simulink model "GPCA_INFUSION_MGR"  (Simulink 8.5)
settings: Solver=ode45  StartTime=0.0  StopTime=10.0  RelTol=1e-3
libraries: simulink x4
settings Model: Creator=bourbouh  LastModifiedBy=Teme
settings DataIOCC: LimitDataPoints=off  SaveFormat=Dataset  SignalLoggingSaveFormat=Dataset
settings OptimizationCC: ExpressionDepthLimit=128
settings DebuggingCC: UnderspecifiedInitializationDetection=Simplified  MergeDetectMultiDrivingBlocksExec=error  FcnCallInpInsideContextMsg=EnableAllAsError  StateNameClashWarn=none
settings HardwareCC: ProdBitPerInt=16  ProdBitPerPointer=16  ProdIntDivRoundTo=Zero  ProdWordSize=8  ProdShiftRightIntArith=off  ProdHWDeviceType=Intel->8051 Compatible  TargetBitPerPointer=64  TargetLargestAtomicFloat=Float  TargetIntDivRoundTo=Zero  TargetEndianess=LittleEndian  TargetWordSize=64  TargetHWDeviceType=Intel->x86-64 (Windows64)  ProdEqTarget=off
settings ModelReferenceCC: PropagateSignalLabelsOutOfModel=on
settings GRTTargetCC: CombineOutputUpdateFcns=on  GRTInterface=off
settings ConfigComp: CovMetricSettings=dw  CovHtmlReporting=on  CovSaveCumulativeToWorkspaceVar=on  CovSaveSingleToWorkspaceVar=on  CovExternalEMLEnable=off

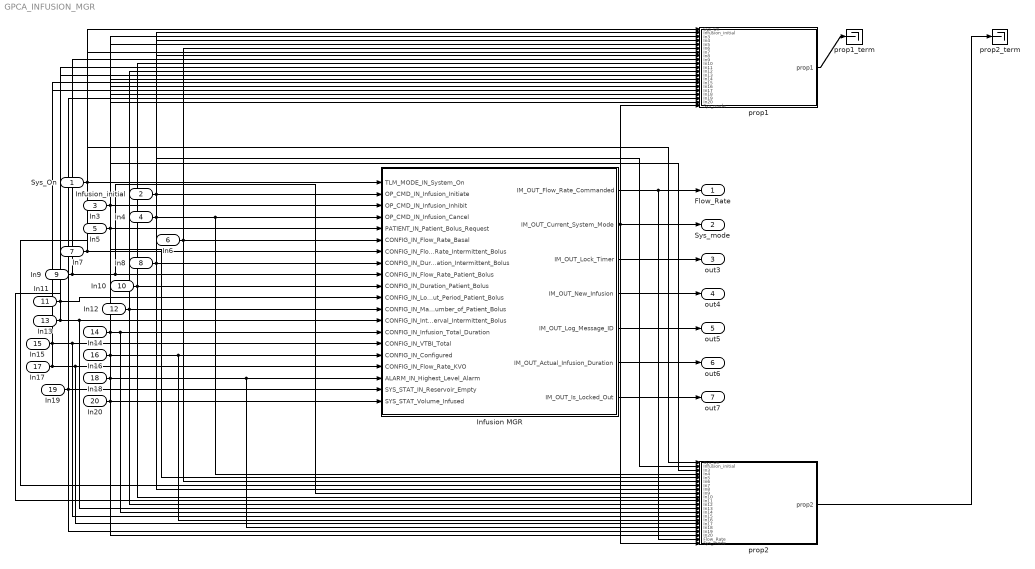
== system GPCA_INFUSION_MGR ==
  Sys_On : Inport
  Infusion_initial : Inport  Port=2
  In3 : Inport  Port=3
  In4 : Inport  Port=4
  In5 : Inport  Port=5
  In6 : Inport  Port=6
  In7 : Inport  Port=7
  In8 : Inport  Port=8
  In9 : Inport  Port=9
  In10 : Inport  Port=10
  In11 : Inport  Port=11
  In12 : Inport  Port=12
  In13 : Inport  Port=13
  In14 : Inport  Port=14
  In15 : Inport  Port=15
  In16 : Inport  Port=16
  In17 : Inport  Port=17
  In18 : Inport  Port=18
  In19 : Inport  Port=19
  In20 : Inport  Port=20
  Infusion MGR : Stateflow chart  TreatAsAtomicUnit=on
  prop1 : Subsystem  TreatAsAtomicUnit=on  mask(Observer){AnnotationType=ensures, ObserverType=[]}
      mask prompts: AnnotationType "Type of annotation (pre/post...)"; ObserverType "Observer type"
      mask help:
      | Set an observer for the system.
      | The annotation type parameter sets the type of observer:
      | - requires : pre-condition
      | - ensures : post-condition
      | - assert : an assertion
      | - observer : the observer computes a special type of properties
      mask TypeOptions AnnotationType: ensures | requires | assert | observer
      mask Callback AnnotationType:
      | paramStr = get_param(gcb, 'MaskValues');
      | if strcmp(paramStr{1}(1),'o')
      | set_param(gcb,'MaskVisibilities',{'on';'on'});
      | paramStr{2} = 'ellipsoid';
      | set_param(gcb,'MaskValues',paramStr);
      | else
      | set_param(gcb,'MaskVisibilities',{'on';'off'});
      | end
      | clear paramStr;
      mask Callback ObserverType:
      | paramStr = get_param(gcb, 'MaskValues');
      | if strcmp(paramStr{1}(1),'o')
      | set_param(gcb,'MaskVisibilities',{'on';'on'});
      | paramStr{2} = 'ellipsoid';
      | set_param(gcb,'MaskValues',paramStr);
      | else
      | set_param(gcb,'MaskVisibilities',{'on';'off'});
      | end
      | clear paramStr;
      mask Display:
      | color('black')
      | text(0.5, 0.5, ['Property: ''' get_param(gcb,'name') ''''], 'horizontalAlignment', 'center');
      | text(0.99, 0.03, '{\bf\fontsize{12}SAFE}', 'hor', 'right', 'ver', 'bottom', 'texmode', 'on');
  prop1_term : Terminator
  prop2 : Subsystem  TreatAsAtomicUnit=on  mask(Observer){AnnotationType=ensures, ObserverType=[]}
      mask prompts: AnnotationType "Type of annotation (pre/post...)"; ObserverType "Observer type"
      mask help:
      | Set an observer for the system.
      | The annotation type parameter sets the type of observer:
      | - requires : pre-condition
      | - ensures : post-condition
      | - assert : an assertion
      | - observer : the observer computes a special type of properties
      mask TypeOptions AnnotationType: ensures | requires | assert | observer
      mask Callback AnnotationType:
      | paramStr = get_param(gcb, 'MaskValues');
      | if strcmp(paramStr{1}(1),'o')
      | set_param(gcb,'MaskVisibilities',{'on';'on'});
      | paramStr{2} = 'ellipsoid';
      | set_param(gcb,'MaskValues',paramStr);
      | else
      | set_param(gcb,'MaskVisibilities',{'on';'off'});
      | end
      | clear paramStr;
      mask Callback ObserverType:
      | paramStr = get_param(gcb, 'MaskValues');
      | if strcmp(paramStr{1}(1),'o')
      | set_param(gcb,'MaskVisibilities',{'on';'on'});
      | paramStr{2} = 'ellipsoid';
      | set_param(gcb,'MaskValues',paramStr);
      | else
      | set_param(gcb,'MaskVisibilities',{'on';'off'});
      | end
      | clear paramStr;
      mask Display:
      | color('black')
      | text(0.5, 0.5, ['Property: ''' get_param(gcb,'name') ''''], 'horizontalAlignment', 'center');
      | text(0.99, 0.03, '{\bf\fontsize{12}TIMEOUT}', 'hor', 'right', 'ver', 'bottom', 'texmode', 'on');
  prop2_term : Terminator
  Flow_Rate : Outport
  Sys_mode : Outport  Port=2
  out3 : Outport  Port=3
  out4 : Outport  Port=4
  out5 : Outport  Port=5
  out6 : Outport  Port=6
  out7 : Outport  Port=7
  wires:
  Sys_On/1 -> Infusion MGR/1(TLM_MODE_IN_System_On), prop1/1(Sys_On), prop2/1(Sys_On)
  Infusion_initial/1 -> Infusion MGR/2(OP_CMD_IN_Infusion_Initiate), prop1/2(Infusion_initial), prop2/2(Infusion_initial)
  In3/1 -> Infusion MGR/3(OP_CMD_IN_Infusion_Inhibit), prop1/3(In3), prop2/3(In3)
  In4/1 -> Infusion MGR/4(OP_CMD_IN_Infusion_Cancel), prop2/4(In4), prop1/4(In4)
  In5/1 -> Infusion MGR/5(PATIENT_IN_Patient_Bolus_Request), prop1/5(In5), prop2/5(In5)
  In6/1 -> Infusion MGR/6(CONFIG_IN_Flow_Rate_Basal), prop1/6(In6), prop2/6(In6)
  In7/1 -> Infusion MGR/7(CONFIG_IN_Flow_Rate_Intermittent_Bolus), prop1/7(In7), prop2/7(In7)
  In8/1 -> Infusion MGR/8(CONFIG_IN_Duration_Intermittent_Bolus), prop1/8(In8), prop2/8(In8)
  In9/1 -> Infusion MGR/9(CONFIG_IN_Flow_Rate_Patient_Bolus), prop2/9(In9), prop1/9(In9)
  In10/1 -> Infusion MGR/10(CONFIG_IN_Duration_Patient_Bolus), prop1/10(In10), prop2/10(In10)
  In11/1 -> Infusion MGR/11(CONFIG_IN_Lockout_Period_Patient_Bolus), prop1/11(In11), prop2/11(In11)
  In12/1 -> Infusion MGR/12(CONFIG_IN_Max_Number_of_Patient_Bolus), prop1/12(In12), prop2/12(In12)
  In13/1 -> Infusion MGR/13(CONFIG_IN_Interval_Intermittent_Bolus), prop2/13(In13), prop1/13(In13)
  In14/1 -> Infusion MGR/14(CONFIG_IN_Infusion_Total_Duration), prop2/14(In14), prop1/14(In14)
  In15/1 -> Infusion MGR/15(CONFIG_IN_VTBI_Total), prop2/15(In15), prop1/15(In15)
  In16/1 -> Infusion MGR/16(CONFIG_IN_Configured), prop2/16(In16), prop1/16(In16)
  In17/1 -> Infusion MGR/17(CONFIG_IN_Flow_Rate_KVO), prop2/17(In17), prop1/17(In17)
  In18/1 -> Infusion MGR/18(ALARM_IN_Highest_Level_Alarm), prop2/18(In18), prop1/18(In18)
  In19/1 -> Infusion MGR/19(SYS_STAT_IN_Reservoir_Empty), prop1/19(In19), prop2/19(In19)
  In20/1 -> Infusion MGR/20(SYS_STAT_Volume_Infused), prop1/20(In20), prop2/20(In20)
  Infusion MGR/2(IM_OUT_Current_System_Mode) -> Sys_mode/1, prop1/21(Sys_mode), prop2/22(Sys_mode)
  Infusion MGR/3(IM_OUT_Lock_Timer) -> out3/1
  Infusion MGR/1(IM_OUT_Flow_Rate_Commanded) -> Flow_Rate/1, prop2/21(Flow_Rate)
  Infusion MGR/4(IM_OUT_New_Infusion) -> out4/1
  Infusion MGR/5(IM_OUT_Log_Message_ID) -> out5/1
  Infusion MGR/6(IM_OUT_Actual_Infusion_Duration) -> out6/1
  Infusion MGR/7(IM_OUT_Is_Locked_Out) -> out7/1
  prop1/1(prop1) -> prop1_term/1
  prop2/1(prop2) -> prop2_term/1

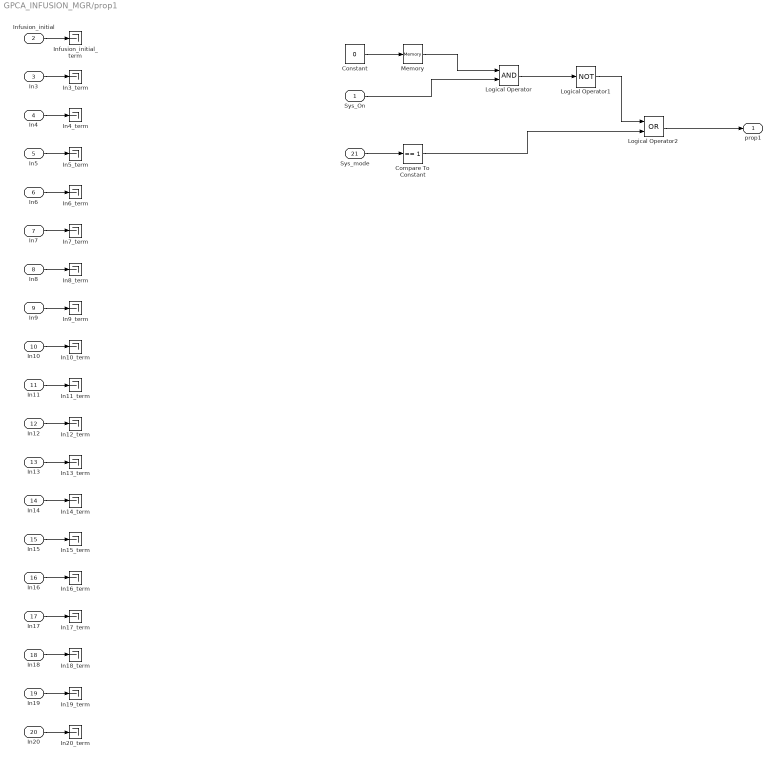
== system GPCA_INFUSION_MGR/prop1 ==
  Sys_On : Inport
  Infusion_initial : Inport  Port=2
  In3 : Inport  Port=3
  In4 : Inport  Port=4
  In5 : Inport  Port=5
  In6 : Inport  Port=6
  In7 : Inport  Port=7
  In8 : Inport  Port=8
  In9 : Inport  Port=9
  In10 : Inport  Port=10
  In11 : Inport  Port=11
  In12 : Inport  Port=12
  In13 : Inport  Port=13
  In14 : Inport  Port=14
  In15 : Inport  Port=15
  In16 : Inport  Port=16
  In17 : Inport  Port=17
  In18 : Inport  Port=18
  In19 : Inport  Port=19
  In20 : Inport  Port=20
  Sys_mode : Inport  Port=21
  Compare To Constant : simulink/Logic and Bit Operations/Compare To Constant  relop===  const=1  OutDataTypeStr=boolean
  Constant : Constant  Value=0
  In10_term : Terminator
  In11_term : Terminator
  In12_term : Terminator
  In13_term : Terminator
  In14_term : Terminator
  In15_term : Terminator
  In16_term : Terminator
  In17_term : Terminator
  In18_term : Terminator
  In19_term : Terminator
  In20_term : Terminator
  In3_term : Terminator
  In4_term : Terminator
  In5_term : Terminator
  In6_term : Terminator
  In7_term : Terminator
  In8_term : Terminator
  In9_term : Terminator
  Infusion_initial_term : Terminator
  Logical Operator : Logic  AllPortsSameDT=off  OutDataTypeStr=boolean
  Logical Operator1 : Logic  Operator=NOT  AllPortsSameDT=off  OutDataTypeStr=boolean
  Logical Operator2 : Logic  Operator=OR  AllPortsSameDT=off  OutDataTypeStr=boolean
  Memory : Memory  X0=1
  prop1 : Outport
  wires:
  Sys_On/1 -> Logical Operator/2
  Infusion_initial/1 -> Infusion_initial_term/1
  In3/1 -> In3_term/1
  In4/1 -> In4_term/1
  In5/1 -> In5_term/1
  In6/1 -> In6_term/1
  In7/1 -> In7_term/1
  In8/1 -> In8_term/1
  In9/1 -> In9_term/1
  In10/1 -> In10_term/1
  In11/1 -> In11_term/1
  In12/1 -> In12_term/1
  In13/1 -> In13_term/1
  In14/1 -> In14_term/1
  In15/1 -> In15_term/1
  In16/1 -> In16_term/1
  In17/1 -> In17_term/1
  In18/1 -> In18_term/1
  In19/1 -> In19_term/1
  In20/1 -> In20_term/1
  Sys_mode/1 -> Compare To Constant/1
  Constant/1 -> Memory/1
  Memory/1 -> Logical Operator/1
  Logical Operator/1 -> Logical Operator1/1
  Logical Operator1/1 -> Logical Operator2/1
  Compare To Constant/1 -> Logical Operator2/2
  Logical Operator2/1 -> prop1/1

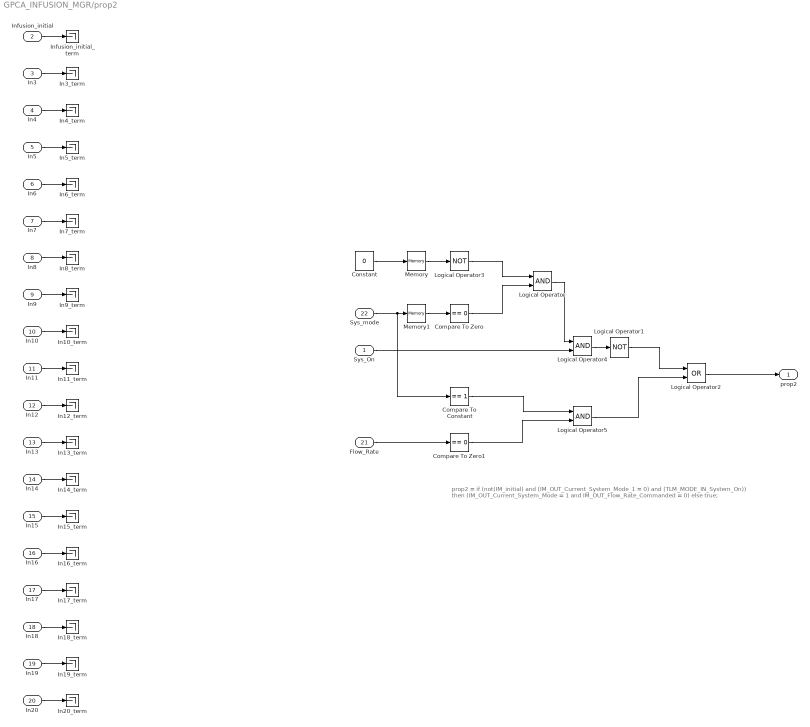
== system GPCA_INFUSION_MGR/prop2 ==
  note: prop2 =	if (not(IM_initial) and (IM_OUT_Current_System_Mode_1 = 0) and (TLM_MODE_IN_System_On))
      | 		then (IM_OUT_Current_System_Mode = 1 and IM_OUT_Flow_Rate_Commanded = 0) else true;
  Sys_On : Inport
  Infusion_initial : Inport  Port=2
  In3 : Inport  Port=3
  In4 : Inport  Port=4
  In5 : Inport  Port=5
  In6 : Inport  Port=6
  In7 : Inport  Port=7
  In8 : Inport  Port=8
  In9 : Inport  Port=9
  In10 : Inport  Port=10
  In11 : Inport  Port=11
  In12 : Inport  Port=12
  In13 : Inport  Port=13
  In14 : Inport  Port=14
  In15 : Inport  Port=15
  In16 : Inport  Port=16
  In17 : Inport  Port=17
  In18 : Inport  Port=18
  In19 : Inport  Port=19
  In20 : Inport  Port=20
  Flow_Rate : Inport  Port=21
  Sys_mode : Inport  Port=22
  Compare To Constant : simulink/Logic and Bit Operations/Compare To Constant  relop===  const=1  OutDataTypeStr=boolean
  Compare To Zero : simulink/Logic and Bit Operations/Compare To Zero  relop===  OutDataTypeStr=boolean
  Compare To Zero1 : simulink/Logic and Bit Operations/Compare To Zero  relop===  OutDataTypeStr=boolean
  Constant : Constant  Value=0
  In10_term : Terminator
  In11_term : Terminator
  In12_term : Terminator
  In13_term : Terminator
  In14_term : Terminator
  In15_term : Terminator
  In16_term : Terminator
  In17_term : Terminator
  In18_term : Terminator
  In19_term : Terminator
  In20_term : Terminator
  In3_term : Terminator
  In4_term : Terminator
  In5_term : Terminator
  In6_term : Terminator
  In7_term : Terminator
  In8_term : Terminator
  In9_term : Terminator
  Infusion_initial_term : Terminator
  Logical Operator : Logic  AllPortsSameDT=off  OutDataTypeStr=boolean
  Logical Operator1 : Logic  Operator=NOT  AllPortsSameDT=off  OutDataTypeStr=boolean
  Logical Operator2 : Logic  Operator=OR  AllPortsSameDT=off  OutDataTypeStr=boolean
  Logical Operator3 : Logic  Operator=NOT  AllPortsSameDT=off  OutDataTypeStr=boolean
  Logical Operator4 : Logic  AllPortsSameDT=off  OutDataTypeStr=boolean
  Logical Operator5 : Logic  AllPortsSameDT=off  OutDataTypeStr=boolean
  Memory : Memory  X0=1
  Memory1 : Memory
  prop2 : Outport
  wires:
  Sys_On/1 -> Logical Operator4/2
  Infusion_initial/1 -> Infusion_initial_term/1
  In3/1 -> In3_term/1
  In4/1 -> In4_term/1
  In5/1 -> In5_term/1
  In6/1 -> In6_term/1
  In7/1 -> In7_term/1
  In8/1 -> In8_term/1
  In9/1 -> In9_term/1
  In10/1 -> In10_term/1
  In11/1 -> In11_term/1
  In12/1 -> In12_term/1
  In13/1 -> In13_term/1
  In14/1 -> In14_term/1
  In15/1 -> In15_term/1
  In16/1 -> In16_term/1
  In17/1 -> In17_term/1
  In18/1 -> In18_term/1
  In19/1 -> In19_term/1
  In20/1 -> In20_term/1
  Flow_Rate/1 -> Compare To Zero1/1
  Compare To Zero/1 -> Logical Operator/2
  Sys_mode/1 -> Compare To Constant/1, Memory1/1
  Constant/1 -> Memory/1
  Logical Operator/1 -> Logical Operator4/1
  Logical Operator1/1 -> Logical Operator2/1
  Logical Operator2/1 -> prop2/1
  Memory/1 -> Logical Operator3/1
  Logical Operator3/1 -> Logical Operator/1
  Logical Operator4/1 -> Logical Operator1/1
  Compare To Constant/1 -> Logical Operator5/1
  Compare To Zero1/1 -> Logical Operator5/2
  Logical Operator5/1 -> Logical Operator2/2
  Memory1/1 -> Compare To Zero/1

== stateflow chart Infusion MGR ==
  state NOT_ON
    entry: IM_OUT_Current_System_Mode=0;
    IM_OUT_Flow_Rate_Commanded=0;
    during: IM_OUT_Current_System_Mode=0;
    IM_OUT_Flow_Rate_Commanded=0;
    exit:IM_OUT_Current_System_Mode=0;
    IM_OUT_Flow_Rate_Commanded=0;
  state Infusion_Manager
    state THERAPY
      during: IM_OUT_New_Infusion=0;
      exit:TherapyExitOperations();
      state ACTIVE
        state Arbiter [parallel]
          settings: executionOrder=4
          state Patient_Bolus
            entry: IM_OUT_Flow_Rate_Commanded=CONFIG_IN_Flow_Rate_Patient_Bolus;
            IM_OUT_Current_System_Mode=4;
            during: IM_OUT_Flow_Rate_Commanded=CONFIG_IN_Flow_Rate_Patient_Bolus;
            IM_OUT_Current_System_Mode=4;
          state Intermittent_Bolus
            entry: IM_OUT_Flow_Rate_Commanded=CONFIG_IN_Flow_Rate_Intermittent_Bolus;
            IM_OUT_Current_System_Mode=3;
            during: IM_OUT_Flow_Rate_Commanded=CONFIG_IN_Flow_Rate_Intermittent_Bolus;
            IM_OUT_Current_System_Mode=3;
          state Basal
            entry:IM_OUT_Flow_Rate_Commanded=CONFIG_IN_Flow_Rate_Basal;
            IM_OUT_Current_System_Mode=2;
            during:IM_OUT_Flow_Rate_Commanded=CONFIG_IN_Flow_Rate_Basal;
            IM_OUT_Current_System_Mode=2;
          (default) -> (junction 54)
          (junction 54) -> Patient_Bolus [order 1] : [in(PATIENT.ON)]
          (junction 54) -> Intermittent_Bolus [order 2] : [in(INTERMITTENT.ON)]
          (junction 54) -> Basal [order 3]
          (junction 55) -> (junction 54)
          Patient_Bolus -> (junction 56)
          Intermittent_Bolus -> (junction 56)
          Basal -> (junction 56)
          (junction 56) -> (junction 55) : {IM_OUT_Actual_Infusion_Duration++}
        state BASAL [parallel]
          settings: executionOrder=1
          state ON
          state OFF
          (default) -> Infusion_Manager.THERAPY.ACTIVE.BASAL.ON
          Infusion_Manager.THERAPY.ACTIVE.BASAL.OFF -> Infusion_Manager.THERAPY.ACTIVE.BASAL.ON : [OP_CMD_IN_Infusion_Initiate]
          Infusion_Manager.THERAPY.ACTIVE.BASAL.ON -> Infusion_Manager.THERAPY.ACTIVE.BASAL.OFF : [IM_OUT_Actual_Infusion_Duration >= Step_Scaling_Factor(CONFIG_IN_Infusion_Total_Duration-1,step_size)]
        state PATIENT [parallel]
          settings: executionOrder=2
          state ON
            entry:number_pbolus++;
            inPatientBolus=1;
            pbolus_timer++;
            IM_OUT_Is_Locked_Out=false;
            during: pbolus_timer++;
            exit: pbolus_timer++;
          state OFF
            entry:pbolus_timer=0;
            inPatientBolus=0;
            IM_OUT_Is_Locked_Out=false;
          state LOCKOUT
            entry:IM_OUT_Lock_Timer++;
            IM_OUT_Is_Locked_Out=true;
            during:IM_OUT_Is_Locked_Out=true;
            IM_OUT_Lock_Timer++;
          (default) -> Infusion_Manager.THERAPY.ACTIVE.PATIENT.OFF [order 2]
          Infusion_Manager.THERAPY.ACTIVE.PATIENT.OFF -> Infusion_Manager.THERAPY.ACTIVE.PATIENT.ON : [PATIENT_IN_Patient_Bolus_Request  && ALARM_IN_Highest_Level_Alarm < 2 && number_pbolus<CONFIG_IN_Max_Number_of_Patient_Bolus ]
          Infusion_Manager.THERAPY.ACTIVE.PATIENT.ON -> LOCKOUT : [pbolus_timer >= Step_Scaling_Factor(CONFIG_IN_Duration_Patient_Bolus-1, step_size) || ALARM_IN_Highest_Level_Alarm == 2]{IM_OUT_Lock_Timer=0;}
          LOCKOUT -> Infusion_Manager.THERAPY.ACTIVE.PATIENT.OFF : [IM_OUT_Lock_Timer >= Step_Scaling_Factor(CONFIG_IN_Lockout_Period_Patient_Bolus-1,step_size)]
          (default) -> LOCKOUT [order 1] : [inPatientBolus]
        state INTERMITTENT [parallel]
          entry: sbolusInter_timer++;
          during : sbolusInter_timer++;
          settings: executionOrder=3
          state ON
            during: sbolus_timer++;
            sbolus_req=0;
            exit: sbolus_timer++;
            sbolus_req=0;
          state OFF
            entry:sbolus_timer=0;
            sbolus_req= sbolus_trigger(sbolusInter_timer, CONFIG_IN_Interval_Intermittent_Bolus, step_size);
            sbolus_trigger2(sbolus_req);
            during: sbolus_req= sbolus_trigger(sbolusInter_timer, CONFIG_IN_Interval_Intermittent_Bolus, step_size);
            sbolus_trigger2(sbolus_req);
            state sbolus_trigger2(sb) [function]
              (default) -> (junction 78) : [sb==1]{sbolusInter_timer=0;}
          (default) -> Infusion_Manager.THERAPY.ACTIVE.INTERMITTENT.OFF
          Infusion_Manager.THERAPY.ACTIVE.INTERMITTENT.OFF -> Infusion_Manager.THERAPY.ACTIVE.INTERMITTENT.ON : [sbolus_req  && ALARM_IN_Highest_Level_Alarm < 2 ]
          Infusion_Manager.THERAPY.ACTIVE.INTERMITTENT.ON -> Infusion_Manager.THERAPY.ACTIVE.INTERMITTENT.OFF : [sbolus_timer >= Step_Scaling_Factor(CONFIG_IN_Duration_Intermittent_Bolus-1,step_size) || ALARM_IN_Highest_Level_Alarm == 2]
        state sb= sbolus_trigger(sbolusInter_timer, CONFIG_IN_Interval_Intermittent_Bolus, step_size) [function]
          (default) -> (junction 84) : {sb = 0;}
          (junction 84) -> (junction 85) [order 1] : [sbolusInter_timer > Step_Scaling_Factor(CONFIG_IN_Interval_Intermittent_Bolus, step_size) || sbolusInter_timer < Step_Scaling_Factor(CONFIG_IN_Interval_Intermittent_Bolus, step_size) ]{sb = 0;}
          (junction 84) -> (junction 86) [order 2] : [sbolusInter_timer == Step_Scaling_Factor(CONFIG_IN_Interval_Intermittent_Bolus, step_size)] {sb = 1;}
      state PAUSED
        state Arbiter [parallel]
          settings: executionOrder=3
          state Paused_NoKVO
            entry: IM_OUT_Flow_Rate_Commanded =0;
            IM_OUT_Current_System_Mode=6;
            during: IM_OUT_Flow_Rate_Commanded =0;
            IM_OUT_Current_System_Mode=6;
            exit: IM_OUT_Flow_Rate_Commanded =0;
            IM_OUT_Current_System_Mode=6;
          state Paused_KVO
            entry: IM_OUT_Flow_Rate_Commanded =CONFIG_IN_Flow_Rate_KVO;
            IM_OUT_Current_System_Mode=7;
            during: IM_OUT_Flow_Rate_Commanded =CONFIG_IN_Flow_Rate_KVO;
            IM_OUT_Current_System_Mode=7;
            exit: IM_OUT_Flow_Rate_Commanded =CONFIG_IN_Flow_Rate_KVO;
            IM_OUT_Current_System_Mode=7;
          state Manual_Paused_KVO
            entry:IM_OUT_Flow_Rate_Commanded=CONFIG_IN_Flow_Rate_KVO;
            IM_OUT_Current_System_Mode=8;
            during:IM_OUT_Flow_Rate_Commanded=CONFIG_IN_Flow_Rate_KVO;
            IM_OUT_Current_System_Mode=8;
            exit:IM_OUT_Flow_Rate_Commanded=CONFIG_IN_Flow_Rate_KVO;
            IM_OUT_Current_System_Mode=8;
          (default) -> (junction 90)
          (junction 90) -> Paused_NoKVO [order 1] : [in(Alarm_Paused.ON) && ALARM_IN_Highest_Level_Alarm == 4]
          (junction 90) -> Paused_KVO [order 2] : [in(Alarm_Paused.ON) && ALARM_IN_Highest_Level_Alarm == 3]
          (junction 90) -> Manual_Paused_KVO [order 3]
          (junction 91) -> (junction 90)
          Paused_NoKVO -> (junction 92)
          Paused_KVO -> (junction 92)
          Manual_Paused_KVO -> (junction 92)
          (junction 92) -> (junction 91)
        state Alarm_Paused [parallel]
          settings: executionOrder=1
          state OFF
          state ON
          (default) -> Infusion_Manager.THERAPY.PAUSED.Alarm_Paused.OFF [order 2]
          (default) -> Infusion_Manager.THERAPY.PAUSED.Alarm_Paused.ON [order 1] : [ALARM_IN_Highest_Level_Alarm >= 3]
          Infusion_Manager.THERAPY.PAUSED.Alarm_Paused.OFF -> Infusion_Manager.THERAPY.PAUSED.Alarm_Paused.ON : [ALARM_IN_Highest_Level_Alarm >= 3]
          Infusion_Manager.THERAPY.PAUSED.Alarm_Paused.ON -> Infusion_Manager.THERAPY.PAUSED.Alarm_Paused.OFF : [OP_CMD_IN_Infusion_Initiate && ALARM_IN_Highest_Level_Alarm < 3]
        state Manual_Paused [parallel]
          settings: executionOrder=2
          state OFF
          state ON
          (default) -> Infusion_Manager.THERAPY.PAUSED.Manual_Paused.OFF [order 2]
          (default) -> Infusion_Manager.THERAPY.PAUSED.Manual_Paused.ON [order 1] : [OP_CMD_IN_Infusion_Inhibit]
          Infusion_Manager.THERAPY.PAUSED.Manual_Paused.OFF -> Infusion_Manager.THERAPY.PAUSED.Manual_Paused.ON : [OP_CMD_IN_Infusion_Inhibit]
          Infusion_Manager.THERAPY.PAUSED.Manual_Paused.ON -> Infusion_Manager.THERAPY.PAUSED.Manual_Paused.OFF : [OP_CMD_IN_Infusion_Initiate && !OP_CMD_IN_Infusion_Inhibit]
      state TherapyExitOperations [function]
        (default) -> (junction 110) : {IM_OUT_Flow_Rate_Commanded=0;
            | IM_OUT_New_Infusion=0;
            | IM_OUT_Is_Locked_Out=false;}
      (default) -> PAUSED [order 1] : [OP_CMD_IN_Infusion_Inhibit || ALARM_IN_Highest_Level_Alarm >= 3]
      (default) -> ACTIVE [order 2]
      ACTIVE -> PAUSED : [OP_CMD_IN_Infusion_Inhibit || ALARM_IN_Highest_Level_Alarm >= 3]
      PAUSED -> ACTIVE : [OP_CMD_IN_Infusion_Initiate && ALARM_IN_Highest_Level_Alarm < 3 && !OP_CMD_IN_Infusion_Inhibit]
    state IDLE
      entry:IM_OUT_Current_System_Mode=1;
      IM_OUT_Flow_Rate_Commanded=0;
      resetAllInfusionDetails();
      during :IM_OUT_Current_System_Mode=1;
      IM_OUT_Flow_Rate_Commanded=0;
      exit:IM_OUT_Current_System_Mode=1;
      IM_OUT_Flow_Rate_Commanded=0;
      resetAllInfusionDetails();
    state resetAllInfusionDetails [function]
      (default) -> (junction 112) : {/*resetForNewInfusion();*/
          | IM_OUT_Lock_Timer=0;
          | inPatientBolus=0;
          | number_pbolus=0;
          | IM_OUT_Is_Locked_Out=false;}
    note: From Therapy - you exit, when
        | 1. Infusion complete
        | 2. Infusion is cancelled : Either Volume or Time is reached
        | 3. No Configuration is avaliable
        | 4. Infsuion is tried to be initiated when there no reservoir volume.
        | -- More conditions may need to be added here.
    state sbolus_dur_timer_fun [function]
      (default) -> (junction 114) : {sbolus_dur_timer=0;
          | sbolus_timer=0;
          | pbolus_timer =0;
          | number_pbolus=0;
          | pbolus_dur_timer=0;
          | sbolusInter_timer=0;
          | paused_KVO_timer=0;
          | IM_OUT_Flow_Rate_Commanded=0;
          | IM_OUT_Actual_Infusion_Duration=0;
          | IM_OUT_Is_Locked_Out=false;
          | writeLog(1);}
    (default) -> IDLE
    THERAPY -> (junction 43) [order 1] : [OP_CMD_IN_Infusion_Initiate && CONFIG_IN_Configured ==1 && !SYS_STAT_IN_Reservoir_Empty ] {/*resetForNewInfusion();*/}
    (junction 43) -> THERAPY : {IM_OUT_New_Infusion=1;}
    IDLE -> (junction 43) [order 2] : [OP_CMD_IN_Infusion_Initiate && CONFIG_IN_Configured > 0 && !SYS_STAT_IN_Reservoir_Empty]{resetAllInfusionDetails();}
    THERAPY -> IDLE [order 2] : [IM_OUT_Actual_Infusion_Duration >=  Step_Scaling_Factor(CONFIG_IN_Infusion_Total_Duration-1, step_size)  || SYS_STAT_Volume_Infused >= CONFIG_IN_VTBI_Total || (CONFIG_IN_Configured < 1) || (OP_CMD_IN_Infusion_Cancel)]
    IDLE -> IDLE [order 1] : [OP_CMD_IN_Infusion_Cancel]
  state writeLog(logEvent) [function]
    (default) -> (junction 117) : {IM_OUT_Log_Message_ID=logEvent;}
  state returnVal = Step_Scaling_Factor(inputVal, step_size) [function]
    note: This is the operational mode.
    (default) -> (junction 122) : {returnVal=inputVal/step_size;}
  note: step scaling factor returns the scaled time depending upon the step size.
      | If counter has to timeout after 100 seconds and if the step size is 0.1 second
      | the new timeout value = 100/0.1 = 1000 steps.
      | default will be one step = 1 second.
  (default) -> Infusion_Manager [order 1] : [TLM_MODE_IN_System_On]
  (default) -> NOT_ON [order 2]
  NOT_ON -> Infusion_Manager : [TLM_MODE_IN_System_On]
  Infusion_Manager -> NOT_ON : [!TLM_MODE_IN_System_On]
  data: sb function_input boolean; sb function_output boolean; sbolusInter_timer function_input double; CONFIG_IN_Interval_Intermittent_Bolus function_input double; step_size function_input double; logEvent function_input uint8; inputVal function_input double; returnVal function_output double; step_size function_input double; TLM_MODE_IN_System_On input boolean; IM_OUT_Flow_Rate_Commanded output uint8; OP_CMD_IN_Infusion_Initiate input boolean; OP_CMD_IN_Infusion_Inhibit input boolean; OP_CMD_IN_Infusion_Cancel input boolean; sbolus_req local boolean; sbolus_timer local double; pbolus_timer local double; PATIENT_IN_Patient_Bolus_Request input boolean; IM_OUT_Current_System_Mode output uint8; paused_KVO_timer local uint8; CONFIG_IN_Flow_Rate_Basal input uint8; CONFIG_IN_Flow_Rate_Intermittent_Bolus input uint8; CONFIG_IN_Duration_Intermittent_Bolus input double; CONFIG_IN_Flow_Rate_Patient_Bolus input uint8; CONFIG_IN_Duration_Patient_Bolus input double; CONFIG_IN_Lockout_Period_Patient_Bolus input double; sbolus_dur_timer local uint8; pbolus_dur_timer local uint8; IM_OUT_Lock_Timer output double; number_pbolus local uint8; CONFIG_IN_Max_Number_of_Patient_Bolus input uint8; CONFIG_IN_Interval_Intermittent_Bolus input double; CONFIG_IN_Infusion_Total_Duration input double; CONFIG_IN_VTBI_Total input uint8; CONFIG_IN_Configured input uint8; CONFIG_IN_Flow_Rate_KVO input uint8; inPatientBolus local boolean; ALARM_IN_Highest_Level_Alarm input uint8; sbolusInter_timer local double; IM_OUT_New_Infusion output boolean; IM_OUT_Log_Message_ID output uint8; SYS_STAT_IN_Reservoir_Empty input boolean; SYS_STAT_Volume_Infused input uint8; IM_OUT_Actual_Infusion_Duration output double; step_size parameter double; IM_OUT_Is_Locked_Out output boolean
